simulink model "power_KundurTwoAreaSystem_0"  (R2021b)
settings: Solver=FixedStepDiscrete  StartTime=0.0  StopTime=5  MaxStep=1/60  RelTol=1e-4
PreLoadFcn:
  | Ts=50e-6;
  | Tctrl=2*Ts;
  | PSSMODEL=1;
undefined symbols (not defined in the file or in its folder): D1, Delta
libraries: spsGenericPowerSystemStabilizerLib x8, spsThreePhaseVIMeasurementLib x6, spsLoadFlowBusLib x6, spsThreePhaseParallelRLCLoadLib x4, spsThreePhasePISectionLineLib x4, spsSynchronousMachinepuStandardLib x4, spsExcitationSystemLib x4, spsSteamTurbineandGovernorLib x4, spsThreePhaseSeriesRLCLoadLib x4, spsThreePhaseTransformerTwoWindingsLib x4, spsThreePhaseBreakerLib x2, spsDistributedParametersLineLib x2
(part 1 of 2)
settings Model: ARTEMISmethode_block_infos=$$__separator__$$  Creator=The MathWorks, Inc.  LastModifiedBy=Pavel
settings SolverCC: AlgebraicLoopSolver=TrustRegion
settings DataIOCC: SaveOutput=off  SignalLogging=off  DSMLogging=off  SaveTime=off  ReturnWorkspaceOutputs=off  TimeSaveName=t  SignalLoggingName=sigsOut
settings OptimizationCC: BlockReduction=off  BooleanDataType=off  OptimizeBlockIOStorage=off  BufferReuse=off  GlobalBufferReuse=off  ExpressionFolding=off  ExpressionDepthLimit=2147483647  LocalBlockOutputs=off  InitFltsAndDblsToZero=on  LifeSpan=inf  OptimizeDataStoreBuffers=off  BusAssignmentInplaceUpdate=off
settings DebuggingCC: SaveWithParameterizedLinksMsg=none  SignalResolutionControl=TryResolveAllWithWarning  MultiTaskDSMMsg=warning  MultiTaskCondExecSysMsg=none  FcnCallInpInsideContextMsg=warning  UnconnectedOutputMsg=none  StateNameClashWarn=warning  SFUnexpectedBacktrackingDiag=warning  SFNoUnconditionalDefaultTransitionDiag=warning  SFExecutionAtInitializationDiag=none  SFMachineParentedDataDiag=warning  ArithmeticOperatorsInVariantConditions=warning
settings HardwareCC: ProdBitPerPointer=32  ProdBitPerSizeT=32  ProdBitPerPtrDiffT=32  ProdLargestAtomicFloat=None  ProdIntDivRoundTo=Undefined  ProdEndianess=Unspecified  ProdWordSize=32  ProdHWDeviceType=32-bit Generic  TargetBitPerPointer=64  TargetBitPerSizeT=64  TargetBitPerPtrDiffT=64  TargetLongLongMode=on  TargetIntDivRoundTo=Zero  TargetEndianess=LittleEndian  TargetWordSize=64  TargetHWDeviceType=MATLAB Host  ProdEqTarget=off
settings ModelReferenceCC: PropagateSignalLabelsOutOfModel=off
settings SFSimCC: SimUseLocalCustomCode=off  CustomCodeUndefinedFunction=UseInterfaceOnly
settings RTWCC: RTWUseLocalCustomCode=off
settings CodeAppCC: StateflowObjectComments=on
settings GRTTargetCC: TargetFcnLib=ansi_tfl_tmw.mat  TargetLangStandard=C89/C90 (ANSI)  CombineOutputUpdateFcns=off  GRTInterface=on
settings ConfigComp: CovMetricSettings=dw  CovSaveCumulativeToWorkspaceVar=on  CovSaveSingleToWorkspaceVar=on  CovExternalEMLEnable=off  CovSFcnEnable=off
settings SimscapeCC: SimscapeNormalizeSystem=off  SimscapeNominalValues={1, 'bar'; 1, 'cm^3/s'; 1, 'bar*kg/s'; 1, 'kJ/kg'; 1, 'kW'; }

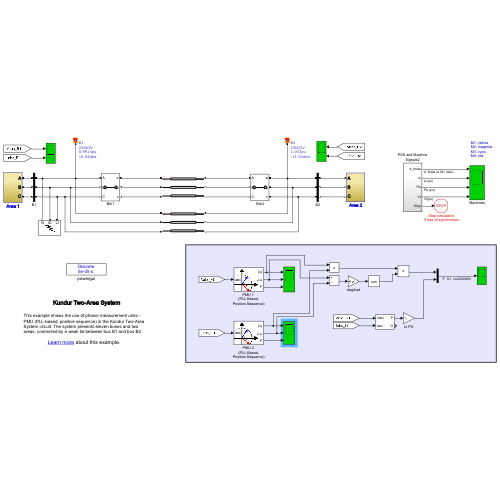
[thumbnail: Simulink's stored preview of the top-level diagram]
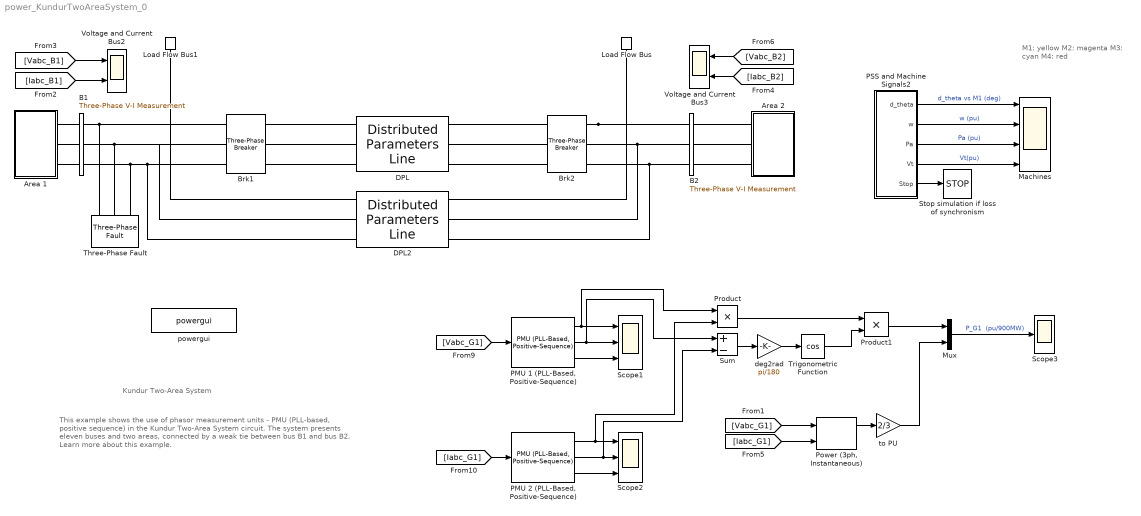
== system power_KundurTwoAreaSystem_0 ==
  note: This example shows the use of phasor measurement units - PMU (PLL-based, positive sequence) in the Kundur Two-Area System circuit. The system presents eleven buses and two areas, connected by a weak tie between bus B1 and bus B2.
      |
      | Learn more about this example.
  note: M1: yellow
      | M2: magenta
      | M3: cyan
      | M4: red
  note: Kundur Two-Area System
  " Brk2" : spsThreePhaseBreakerLib/Three-Phase Breaker  InitialState=closed  SwitchA=on  SwitchB=on  SwitchC=on  SwitchTimes=[2+12]*100  External=off  BreakerResistance=0.001  SnubberResistance=1e6  SnubberCapacitance=0  Measurements=None
      settings: AttributesFormatString=\n
  Area 1 : Subsystem
  Area 2 : Subsystem
  B1 : spsThreePhaseVIMeasurementLib/Three-Phase V-I Measurement  VoltageMeasurement=phase-to-ground  SetLabelV=on  LabelV=Vabc_B1  Vpu=on  VpuLL=off  CurrentMeasurement=yes  SetLabelI=on  LabelI=Iabc_B1  Ipu=off  Pbase=100e6  Vbase=230e3  OutputType=Complex  PhasorSimulation=off  PSBequivalent=0
  B2 : spsThreePhaseVIMeasurementLib/Three-Phase V-I Measurement  VoltageMeasurement=phase-to-ground  SetLabelV=on  LabelV=Vabc_B2  Vpu=off  VpuLL=off  CurrentMeasurement=yes  SetLabelI=on  LabelI=Iabc_B2  Ipu=off  Pbase=100e6  Vbase=500e3  OutputType=Complex  PhasorSimulation=off  PSBequivalent=0
  Brk1 : spsThreePhaseBreakerLib/Three-Phase Breaker  InitialState=closed  SwitchA=off  SwitchB=off  SwitchC=off  SwitchTimes=[2+12]  External=off  BreakerResistance=0.001  SnubberResistance=inf  SnubberCapacitance=0  Measurements=None
      settings: AttributesFormatString=\n
  DPL : spsDistributedParametersLineLib/Distributed Parameters Line  Phases=3  Length=220  Frequency=60  Resistance=[0.0001*529 1.61]  Inductance=[0.001*529/(377) 0.0061]  Capacitance=[0.00175/529/(377) 5.2489e-9]  x1=[-0.00125 5.00401938795932e-05 67714.9475638958 -217904.118381786;-0.0012 4.86656945364756e-05 71810.0841570275 -216589.0762183;-0.00115 4.72739045038167e-05 75879.7069691904 -215197.080987348;-0.0011 4.58653182779878e-05 79922.3700827773 -213728.627258207;-0.00105 4.44404363229678e-05 83936.6371588335 -212184.236765496;-0.001 4.29997648925308e-05 87921.0819473815 -210564.458223802;-0.00095 4.15438158503758e-05 91874.2887941601 -208869.867132729;-0.0009 4.0073106488265e-05 95794.8531436005 -207101.065572422;-0.00085 3.85881593422317e-05 99681.3820378574 -205258.681989653;-0.0008 3.70895020069262e-05 103532.494611721 -203343.370974537;-0.00075 3.55776669481637e-05 107346.822583231 -201355.813027957;-0.0007 3.40531913137418e-05 111123.010739822 -199296.714319788;-0.00065 3.25166167425944e-05 114859.717419823 -197166.806437996;-0.0006 3.096848917235e-05 118555.614989142 -194966.846128709;-0.00055 2.94093586453629e-05 122209.390312972 -192697.61502735;-0.0005 2.78397791132851e-05 125819.745222338 -190359.919380925;-0.00045 2.62603082402508e-05 129385.396975333 -187954.589761565;-0.0004 2.46715072047404e-05 132905.078712866 -185482.48077143;-0.00035 2.30739405001963e-05 136377.539908775 -182944.470739074;-0.0003 2.14681757344618e-05 139801.546814133 -180341.461407377;-0.00025 1.98547834281122e-05 143175.882895589 -177674.377613158;-0.0002 1.82343368117514e-05 146499.349267601 -174944.166958591;-0.00015 1.66074116223463e-05 149770.765118393 -172151.799474521;-0.0001 1.497458589867e-05 152988.968129489 -169298.267275818;-5e-05 1.33364397759271e-05 156152.814888683 -166384.584208886]  x2=[-0.00125 6.64238273339932e-05 -37054.7346638215 -227714.949033752;-0.0012 6.59450869998179e-05 -32756.0754824648 -228372.906194685;-0.00115 6.54429166902368e-05 -28445.7782234611 -228949.723549471;-0.0011 6.49174948239698e-05 -24125.3743149025 -229445.196157652;-0.00105 6.43690080809043e-05 -19796.3987757256 -229859.147980168;-0.001 6.37976513357682e-05 -15460.3896703266 -230191.431941908;-0.00095 6.32036275888925e-05 -11118.8875620942 -230441.929983962;-0.0009 6.25871478940861e-05 -6773.43496605488 -230610.55310557;-0.00085 6.1948431283649e-05 -2425.57580082464 -230697.241395739;-0.0008 6.12877046905515e-05 1923.14515993797 -230701.964054532;-0.00075 6.06052028678062e-05 6271.18283638253 -230624.719404011;-0.0007 5.99011683050607e-05 10616.9923914263 -230465.534888833;-0.00065 5.91758511424429e-05 14959.0297796275 -230224.467066497;-0.0006 5.84295090816871e-05 19295.7522957771 -229901.601587254;-0.00055 5.76624072945735e-05 23625.6191230151 -229497.05316367;-0.0005 5.68748183287145e-05 27947.0918802748 -229010.965529875;-0.00045 5.60670220107194e-05 32258.6351688628 -228443.51139049;-0.0004 5.52393053467737e-05 36558.7171179787 -227794.892359268;-0.00035 5.43919624206668e-05 40845.8099289812 -227065.338887463;-0.0003 5.35252942893056e-05 45118.390418208 -226255.110181951;-0.00025 5.26396088757503e-05 49374.9405581558 -225364.49411313;-0.0002 5.17352208598112e-05 53613.9480168279 -224393.807112651;-0.00015 5.0812451566244e-05 57833.9066950588 -223343.394060983;-0.0001 4.98716288505848e-05 62033.3172616238 -222213.628164881;-5e-05 4.89130869826646e-05 66210.6876859448 -221004.910824788]  x3=[-0.00125 5.68511441714353e-09 -84.0164435730609 325.429221773661;-0.0012 5.94435553554912e-09 -90.1353537591281 323.787794066755;-0.00115 6.20148465273767e-09 -96.2222392831948 322.03132609837;-0.0011 6.4564104119582e-09 -102.274937503818 320.160441933214;-0.00105 6.70904223930233e-09 -108.29129792614 318.175806287519;-0.001 6.95929037588473e-09 -114.269182965951 316.078124292883;-0.00095 7.20706590973406e-09 -120.20646870916 313.868141245729;-0.0009 7.45228080738296e-09 -126.101045666414 311.54664234251;-0.00085 7.69484794514591e-09 -131.950819522587 309.114452400733;-0.0008 7.93468114007387e-09 -137.753711880884 306.572435565903;-0.00075 8.17169518057469e-09 -143.50766100128 303.921495004497;-0.0007 8.40580585668834e-09 -149.210622533051 301.162572583075;-0.00065 8.63692999000634e-09 -154.86057024112 298.296648533634;-0.0006 8.86498546322466e-09 -160.455496725969 295.324741105345;-0.00055 9.08989124931957e-09 -165.993414136859 292.247906202764;-0.0005 9.31156744033618e-09 -171.472354878104 289.067237010682;-0.00045 9.52993527577937e-09 -176.890372308146 285.783863605718;-0.0004 9.74491717059699e-09 -182.245541431192 282.398952554809;-0.00035 9.95643674274547e-09 -187.535959581151 278.913706500733;-0.0003 1.0164418840328e-08 -192.759747097645 275.329363734817;-0.00025 1.03687895682956e-08 -197.915047993843 271.64719775698;-0.0002 1.05694763147019e-08 -203.000030615886 267.86851682326;-0.00015 1.07664077765013e-08 -208.012888293659 263.994663481001;-0.0001 1.09595139848833e-08 -212.951839982699 260.027014091848;-5e-05 1.11487263301314e-08 -217.815130896989 255.966978342738]  x4=[-0.00125 9.68423697480985e-08 -1.92606776170441 -1426.66433970826;-0.0012 9.56520018607397e-08 24.9647096485138 -1426.44709548488;-0.00115 9.44276492725781e-08 51.8466172162664 -1425.72304140067;-0.0011 9.31697469902584e-08 78.7101039277956 -1424.49243470859;-0.00105 9.18787419404718e-08 105.545625314187 -1422.75571263736;-0.001 9.05550928111652e-08 132.343646842472 -1420.51349223604;-0.00095 8.91992698885716e-08 159.094647303204 -1417.76657015487;-0.0009 8.78117548901194e-08 185.789122193297 -1414.51592236219;-0.00085 8.63930407932808e-08 212.417587092931 -1410.76270379768;-0.0008 8.49436316604189e-08 238.970581035323 -1406.50824796203;-0.00075 8.34640424596973e-08 265.43866986816 -1401.75406644312;-0.0007 8.19547988821136e-08 291.81244960551 -1396.50184837903;-0.00065 8.04164371547246e-08 318.082549769014 -1390.75345985782;-0.0006 7.88495038501268e-08 344.239636717173 -1384.51094325456;-0.00055 7.72545556922623e-08 370.274416961545 -1377.77651650567;-0.0005 7.56321593586171e-08 396.177640468675 -1370.55257232091;-0.00045 7.39828912788831e-08 421.940103946593 -1362.84167733325;-0.0004 7.23073374301561e-08 447.552654114697 -1354.64657118697;-0.00035 7.060609312874e-08 473.006190955868 -1345.97016556426;-0.0003 6.88797628186346e-08 498.291670949668 -1336.81554315071;-0.00025 6.71289598567788e-08 523.400110285454 -1327.18595654009;-0.0002 6.53543062951283e-08 548.322588054286 -1317.08482707867;-0.00015 6.35564326596434e-08 573.050249418486 -1306.51574364963;-0.0001 6.17359777262661e-08 597.574308757714 -1295.48246139801;-5e-05 5.98935882939657e-08 621.886052790461 -1283.98890039645]  x5=0.00124486354111605  V1=ones(3,3)  V2=ones(3,3)  I1=ones(3,3)  I2=ones(3,3)  nHarmo=1  Measurements=None  Decoupling=off  VsMag0=0  VrMag0=0  VsAngle0=0  VrAngle0=0  IsMag0=0  IrMag0=0  IsAngle0=0  IrAngle0=0
      settings: SourceProductBaseCode=PS
  DPL2 : spsDistributedParametersLineLib/Distributed Parameters Line  Phases=3  Length=220  Frequency=60  Resistance=[0.0001*529 1.61]  Inductance=[0.001*529/(377) 0.0061]  Capacitance=[0.00175/529/(377) 5.2489e-9]  x1=[-0.00125 5.0041693650628e-05 67715.2009241801 -217904.989560214;-0.0012 4.86670938538175e-05 71810.3538926926 -216589.942466454;-0.00115 4.72752028702947e-05 75879.9929844005 -215197.941997455;-0.0011 4.58665152322987e-05 79922.6722759125 -213729.482724354;-0.00105 4.44415314398394e-05 83936.9554225262 -212185.08638374;-0.001 4.30007577828731e-05 87921.416168554 -210565.301692277;-0.00095 4.15447061614197e-05 91874.6388540653 -208870.704151755;-0.0009 4.00738939036873e-05 95795.2189178637 -207101.89584461;-0.00085 3.85888435822674e-05 99681.7633965208 -205259.505220012;-0.0008 3.70900828284681e-05 103532.89141929 -203344.186870577;-0.00075 3.55781441448486e-05 107347.234698721 -201356.621299794;-0.0007 3.4053564716024e-05 111123.438016811 -199297.514680246;-0.00065 3.25168862178058e-05 114860.159706501 -197167.598602711;-0.0006 3.09686546247475e-05 118556.072128367 -194967.629816229;-0.00055 2.94094200161619e-05 122209.862142324 -192698.389959235;-0.0005 2.78397363806809e-05 125820.23157418 -190360.685281844;-0.00045 2.62601614194262e-05 129385.897676864 -187955.346359398;-0.0004 2.46712563478599e-05 132905.593586191 -185483.227797362;-0.00035 2.30735856963883e-05 136378.068770962 -182945.20792769;-0.0003 2.14677171097865e-05 139802.089477278 -180342.188496756;-0.00025 1.98542211455166e-05 143176.439166888 -177675.09434497;-0.0002 1.82336710710118e-05 146499.918949413 -174944.873078184;-0.00015 1.66066426599974e-05 149771.348008313 -172152.494731014;-0.0001 1.49737139879203e-05 152989.564020418 -169298.951422191;-5e-05 1.33354652265625e-05 156153.423568905 -166385.257002064]  x2=[-0.00125 6.64214580413413e-05 -37054.8247033456 -227714.066792769;-0.0012 6.59426867546337e-05 -32756.1821348863 -228372.025807605;-0.00115 6.54404863453161e-05 -28445.9014508868 -228948.845329093;-0.0011 6.49150352428025e-05 -24125.5140735503 -229444.320416002;-0.00105 6.43665201373679e-05 -19796.55501594 -229858.275028394;-0.001 6.37951359138171e-05 -15460.5623365962 -230190.562090165;-0.00095 6.32010855822443e-05 -11119.0765930715 -230441.063541305;-0.0009 6.25845802059036e-05 -6773.64029457802 -230609.690379841;-0.00085 6.19458388262195e-05 -2425.7973539414 -230696.382693461;-0.0008 6.12850883849629e-05 1922.90746094438 -230701.109680798;-0.00075 6.06025636436193e-05 6270.92907596541 -230623.869662375;-0.0007 5.98985070999794e-05 10616.7226597455 -230464.690081204;-0.00065 5.91731689019807e-05 14958.7441725174 -230223.627493033;-0.0006 5.84268067588311e-05 19295.4509147126 -229900.76754625;-0.00055 5.76596858494463e-05 23625.3020750754 -229496.224951457;-0.0005 5.68720787282325e-05 27946.7592781056 -229010.143440713;-0.00045 5.60642652282497e-05 32258.2871306361 -228442.695716463;-0.0004 5.5236532361788e-05 36558.3537673507 -227794.083390181;-0.00035 5.43891742183934e-05 40845.4313950486 -227064.53691074;-0.0003 5.35224918603794e-05 45117.9968354623 -226254.315482529;-0.00025 5.26367932158611e-05 49374.5320664349 -225363.706973363;-0.0002 5.17323929693495e-05 53613.5247612671 -224393.027812206;-0.00015 5.08096124499458e-05 57833.4688260387 -223342.622876741;-0.0001 4.98687795171746e-05 62032.8649347172 -222212.86537084;-5e-05 4.8910228444497e-05 66210.2210618613 -221004.156691966]  x3=[-0.00125 5.67985394464599e-09 -84.0015107882101 325.431384816722;-0.0012 5.93900034567544e-09 -90.1204643958681 323.79023818478;-0.00115 6.19603664816132e-09 -96.2073986316455 322.034050422975;-0.0011 6.45087152832926e-09 -102.260150836792 320.163445496458;-0.00105 6.70341444455978e-09 -108.27657049727 318.179088022253;-0.001 6.95357566955725e-09 -114.254520007822 316.08168303312;-0.00095 7.20126632222959e-09 -120.191875431451 313.871975727066;-0.0009 7.44639839926732e-09 -126.086527254048 311.550751202575;-0.00085 7.6888848064107e-09 -131.936381133887 309.118834179667;-0.0008 7.9286393893939e-09 -137.73935864574 306.577088706881;-0.00075 8.16557696455519e-09 -143.493398019328 303.92641785428;-0.0007 8.39961334910234e-09 -149.196454871861 301.167763392597;-0.00065 8.6306653910223e-09 -154.846502934394 298.302105458627;-0.0006 8.85865099862476e-09 -160.441534771754 295.330462206988;-0.00055 9.08348916970892e-09 -165.979562495772 292.253889448377;-0.0005 9.30510002034319e-09 -171.458618471566 289.073480274447;-0.00045 9.52340481324757e-09 -176.876756016637 285.790364669433;-0.0004 9.73832598576861e-09 -182.232050092516 282.405709108676;-0.00035 9.9497871774371e-09 -187.522597988715 278.920716144182;-0.0003 1.01577132570985e-08 -192.746519998761 275.336623977355;-0.00025 1.03620303496069e-08 -197.901960088036 271.654706019076;-0.0002 1.0562665862072e-08 -202.987086553225 267.876270437266;-0.00015 1.07595485096518e-08 -208.00009267311 264.002659692093;-0.0001 1.09526083408789e-08 -212.939197350484 260.035250059011;-5e-05 1.11417767625146e-08 -217.802645744975 255.975451139772]  x4=[-0.00125 9.68486646687031e-08 -1.94059700386609 -1426.66653467617;-0.0012 9.5658299002309e-08 24.9502243580123 -1426.44956391594;-0.00115 9.44339463977677e-08 51.8321810239799 -1425.72578241787;-0.0011 9.31760418617297e-08 78.6957219628346 -1424.49544733806;-0.00105 9.18850323216868e-08 105.531302686395 -1422.75899580871;-0.001 9.05613764671816e-08 132.329388640611 -1420.51704478279;-0.00095 8.92055445868362e-08 159.080458593144 -1417.77039081481;-0.0009 8.78180184012618e-08 185.77500801622 -1414.52000977786;-0.00085 8.63992908919053e-08 212.403552463537 -1410.76705651684;-0.0008 8.49498661258954e-08 238.956630940049 -1406.51286443818;-0.00075 8.34702590769497e-08 265.424809263407 -1401.75894503605;-0.0007 8.19609954424075e-08 291.798683415886 -1396.5069873554;-0.00065 8.04226114564516e-08 318.068882885582 -1390.75885739177;-0.0006 7.88556536995869e-08 344.22607399571 -1384.51659742837;-0.00055 7.72606789044433e-08 370.260963220821 -1377.78242531044;-0.0005 7.56382537579707e-08 396.164300488741 -1370.55873365728;-0.00045 7.39889547000985e-08 421.92688246708 -1362.84808901212;-0.0004 7.23133677189284e-08 447.539555833133 -1354.6532309303;-0.00035 7.06120881425364e-08 472.993220526012 -1345.97707100588;-0.0003 6.88857204274552e-08 498.27883297985 -1336.82269183715;-0.00025 6.71348779439135e-08 523.387409336944 -1327.19334593145;-0.0002 6.53601827579091e-08 548.310028639672 -1317.09245454953;-0.00015 6.3562265410191e-08 573.037836000067 -1306.52360649;-0.0001 6.17417646922319e-08 597.562045745918 -1295.49055681425;-5e-05 5.98993274192683e-08 621.873944542278 -1283.99722551229]  x5=0.00124486354111605  V1=ones(3,3)  V2=ones(3,3)  I1=ones(3,3)  I2=ones(3,3)  nHarmo=1  Measurements=None  Decoupling=off  VsMag0=0  VrMag0=0  VsAngle0=0  VrAngle0=0  IsMag0=0  IrMag0=0  IsAngle0=0  IrAngle0=0
      settings: SourceProductBaseCode=PS
  Load Flow Bus : spsLoadFlowBusLib/Load Flow Bus  LConnTagsString=a  Phases=single  Connectors=on one side  ID=B2  Vbase=230e3  Vref=1  Vangle=0  VLF=1.003  VLFb=1  VLFc=1  angleLF=-11.54  angleLFb=0  angleLFc=0
      settings: AttributesFormatString=%<ID>\n%<Vbase>V\n%<VLF>pu\n%<angleLF>deg.  SourceProductBaseCode=PS
  Load Flow Bus1 : spsLoadFlowBusLib/Load Flow Bus  LConnTagsString=a  Phases=single  Connectors=on one side  ID=B1  Vbase=230e3  Vref=1  Vangle=0  VLF=0.9914  VLFb=1  VLFc=1  angleLF=15.04  angleLFb=0  angleLFc=0
      settings: AttributesFormatString=%<ID>\n%<Vbase>V\n%<VLF>pu\n%<angleLF>deg.  SourceProductBaseCode=PS
  Machines : Scope  NumInputPorts=4
  Mux : Mux  Inputs=2
  "PMU 1 (PLL-Based, Positive-Sequence)" : spsPMUPLLBasedPositiveSequenceLib/PMU (PLL-Based, Positive-Sequence)  nominalFrequency=60  samplingRate=64  reportingFactor=1
      settings: SourceProductBaseCode=PS
  "PMU 2 (PLL-Based, Positive-Sequence)" : spsPMUPLLBasedPositiveSequenceLib/PMU (PLL-Based, Positive-Sequence)  nominalFrequency=60  samplingRate=64  reportingFactor=1
      settings: SourceProductBaseCode=PS
  PSS and Machine Signals2 : Subsystem
  "Power (3ph, Instantaneous)" : spsPower3phInstantaneousLib/Power (3ph, Instantaneous)
  Product : Product
  Product1 : Product
  Scope1 : Scope  NumInputPorts=3
  Scope2 : Scope  NumInputPorts=3
  Scope3 : Scope
  Stop simulation if loss of synchronism : Stop
  Sum : Sum  Inputs=+-
  Three-Phase Fault : spsThreePhaseFaultLib/Three-Phase Fault  InitialStates=0  FaultA=on  FaultB=on  FaultC=on  GroundFault=on  SwitchTimes=[2 2.1]  External=off  SwitchStatus=NaN  FaultResistance=0.001  GroundResistance=0.001  SnubberResistance=1e6  SnubberCapacitance=inf  Measurements=None
  Trigonometric Function : Trigonometry  Operator=cos
  Voltage and Current Bus2 : Scope  NumInputPorts=2
  Voltage and Current Bus3 : Scope  NumInputPorts=2
  deg2rad : Gain  Gain=pi/180
  powergui : spspowerguiLib/powergui  Priority=2  SimulationMode=Discrete  SampleTime=Ts  frequency=60  Iterations=50  frequencyindice=60  Pbase=100e6  ErrMax=1e-4  UnitsV=kV  UnitsW=MW  buscounter=0  FunctionMessages=off  echomessages=off  EnableUseOfTLC=off  CurrentSourceSwitches=off  DisableSnubberDevices=off  DisableRonSwitches=off  DisableVfSwitches=off  DisplayEquations=off  AutomaticDiscreteSolvers=off  SolverType=Tustin  Interpol=off  ExternalGateDelay=off  methode=off  Ts=0  x0status=blocks  SPID=off  SwTol=0  HookPort=off  NonlinearTolerance=1e-4  nMaxIteration=100  ContinueOnMaxIteration=off  RestoreLinks=warning  ResistiveCurrentMeasurement=off  Frange=logspace(0,3,50)  Ylog=off  Xlog=off  ShowGrid=off  save=off  variable=ZData  structure=0  ZoomFFT=on  StartTime=0.0  cycles=1  DisplayStyle=1  fundamental=60  FreqAxis=off  MaxFrequency=1000  frequencyindicesteady=1  RmsSteady=1  display=off
  to PU : Gain  Gain=2/3
  wires:
  [Iabc_B1] -> Voltage and Current Bus2/2
  [Vabc_B1] -> Voltage and Current Bus2/1
  [Iabc_B2] -> Voltage and Current Bus3/2
  [Vabc_B2] -> Voltage and Current Bus3/1
  PSS and Machine Signals2/1(d_theta) -> Machines/1  "d_theta vs M1 (deg)"
  PSS and Machine Signals2/2(w) -> Machines/2  "w (pu)"
  PSS and Machine Signals2/3(Pa) -> Machines/3  "Pa (pu)"
  PSS and Machine Signals2/4(Vt) -> Machines/4  "Vt(pu)"
  PSS and Machine Signals2/5(Stop) -> Stop simulation if loss of synchronism/1
  [Iabc_G1] -> "PMU 2 (PLL-Based, Positive-Sequence)"/1
  "PMU 2 (PLL-Based, Positive-Sequence)"/3 -> Scope2/3
  [Vabc_G1] -> "PMU 1 (PLL-Based, Positive-Sequence)"/1
  "PMU 1 (PLL-Based, Positive-Sequence)"/3 -> Scope1/3
  Product/1 -> Product1/1
  [Iabc_G1] -> "Power (3ph, Instantaneous)"/2
  "Power (3ph, Instantaneous)"/1 -> to PU/1
  "PMU 2 (PLL-Based, Positive-Sequence)"/1 -> Product/2, Scope2/1
  [Vabc_G1] -> "Power (3ph, Instantaneous)"/1
  "PMU 2 (PLL-Based, Positive-Sequence)"/2 -> Sum/2, Scope2/2
  deg2rad/1 -> Trigonometric Function/1
  "PMU 1 (PLL-Based, Positive-Sequence)"/1 -> Scope1/1, Product/1
  Trigonometric Function/1 -> Product1/2
  Product1/1 -> Mux/1
  Sum/1 -> deg2rad/1
  to PU/1 -> Mux/2
  "PMU 1 (PLL-Based, Positive-Sequence)"/2 -> Sum/1, Scope1/2
  Mux/1 -> Scope3/1  "P_G1  (pu/900MW)"
  connections:
  " Brk2"/RConn1 -- DPL2/RConn1 -- B2/LConn1 -- Load Flow Bus/LConn1
  " Brk2"/RConn2 -- DPL2/RConn2 -- B2/LConn2
  " Brk2"/RConn3 -- DPL2/RConn3 -- B2/LConn3
  B2/RConn3 -- Area 2/LConn3
  B2/RConn2 -- Area 2/LConn2
  Area 2/LConn1 -- B2/RConn1
  Area 1/RConn3 -- B1/LConn3
  Area 1/RConn2 -- B1/LConn2
  Area 1/RConn1 -- B1/LConn1
  " Brk2"/LConn3 -- DPL/RConn3
  " Brk2"/LConn2 -- DPL/RConn2
  DPL/RConn1 -- " Brk2"/LConn1
  Brk1/RConn3 -- DPL/LConn3
  Brk1/RConn2 -- DPL/LConn2
  Brk1/RConn1 -- DPL/LConn1
  DPL2/LConn3 -- B1/RConn3 -- Three-Phase Fault/LConn3 -- Brk1/LConn3
  DPL2/LConn2 -- Brk1/LConn2 -- Three-Phase Fault/LConn2 -- B1/RConn2
  DPL2/LConn1 -- Brk1/LConn1 -- Load Flow Bus1/LConn1 -- Three-Phase Fault/LConn1 -- B1/RConn1

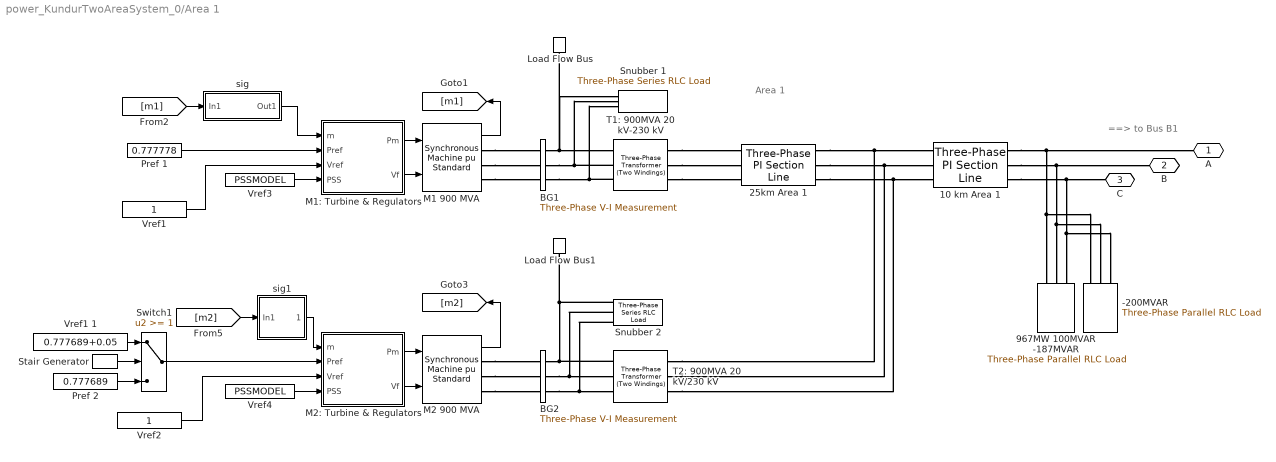
== system power_KundurTwoAreaSystem_0/Area 1 ==
  note: Area 1
  note: ==> to Bus B1
  -200MVAR : spsThreePhaseParallelRLCLoadLib/Three-Phase Parallel RLC Load  LConnTagsString=A|B|C  Configuration=Y (grounded)  NominalVoltage=230e3  Vabc=[1e3 1e3 1e3]  Vabcp=[1e3 1e3 1e3]  NominalFrequency=60  UnbalancedPower=off  ActivePower=0  InductivePower=0  CapacitivePower=200e6  Pabc=[10e3 9e3 11e3]  QLabc=[100 90 110]  QCabc=[100 90 110]  Pabcp=[10e3 9e3 11e3]  QLabcp=[100 90 110]  QCabcp=[100 90 110]  Measurements=None  LoadType=constant Z
  10 km Area 1 : spsThreePhasePISectionLineLib/Three-Phase PI Section Line  LConnTagsString=a|b|c  RConnTagsString=A|B|C  Length=10  Frequency=60  Resistances=[0.0001*529 1.61]  Inductances=[0.001*529/(377) 0.0061]  Capacitances=[0.00175/529/(377) 5.2489e-9]
  25km Area 1 : spsThreePhasePISectionLineLib/Three-Phase PI Section Line  LConnTagsString=a|b|c  RConnTagsString=A|B|C  Length=25  Frequency=60  Resistances=[0.0001*529 1.61]  Inductances=[0.001*529/(377) 0.0061]  Capacitances=[0.00175/529/(377) 5.2489e-9]
  967MW 100MVAR -187MVAR : spsThreePhaseParallelRLCLoadLib/Three-Phase Parallel RLC Load  LConnTagsString=A|B|C  Configuration=Y (grounded)  NominalVoltage=230e3  Vabc=[1e3 1e3 1e3]  Vabcp=[1e3 1e3 1e3]  NominalFrequency=60  UnbalancedPower=off  ActivePower=967e6  InductivePower=100e6  CapacitivePower=187e6  Pabc=[10e3 9e3 11e3]  QLabc=[100 90 110]  QCabc=[100 90 110]  Pabcp=[10e3 9e3 11e3]  QLabcp=[100 90 110]  QCabcp=[100 90 110]  Measurements=None  LoadType=constant Z
  BG1 : spsThreePhaseVIMeasurementLib/Three-Phase V-I Measurement  VoltageMeasurement=phase-to-ground  SetLabelV=on  LabelV=Vabc_G1  Vpu=on  VpuLL=off  CurrentMeasurement=yes  SetLabelI=on  LabelI=Iabc_G1  Ipu=on  Pbase=900e6  Vbase=20e3  OutputType=Complex  PhasorSimulation=off  PSBequivalent=0
  BG2 : spsThreePhaseVIMeasurementLib/Three-Phase V-I Measurement  VoltageMeasurement=no  SetLabelV=on  LabelV=Vabc_G2  Vpu=on  VpuLL=off  CurrentMeasurement=no  SetLabelI=on  LabelI=Iabc_G2  Ipu=on  Pbase=900e6  Vbase=20e3  OutputType=Complex  PhasorSimulation=off  PSBequivalent=0
  Load Flow Bus : spsLoadFlowBusLib/Load Flow Bus  LConnTagsString=a  Phases=single  Connectors=on one side  ID=M1_Area1  Vbase=20e3  Vref=1  Vangle=0  VLF=1  VLFb=1  VLFc=1  angleLF=10.19  angleLFb=0  angleLFc=0
      settings: AttributesFormatString=%<ID>\n%<Vbase>V\n%<VLF>pu\n%<angleLF>deg.  SourceProductBaseCode=PS
  Load Flow Bus1 : spsLoadFlowBusLib/Load Flow Bus  LConnTagsString=a  Phases=single  Connectors=on one side  ID=M2_Area1  Vbase=20e3  Vref=1  Vangle=0  VLF=1  VLFb=1  VLFc=1  angleLF=0  angleLFb=0  angleLFc=0
      settings: AttributesFormatString=%<ID>\n%<Vbase>V\n%<VLF>pu\n%<angleLF>deg.  SourceProductBaseCode=PS
  M1 900 MVA : spsSynchronousMachinepuStandardLib/Synchronous Machine pu Standard  PresetModel=No  MechanicalLoad=Mechanical power Pm  ShowDetailedParameters=on  RotorType=Round  Units=per unit standard parameters  MeasurementBus=off  NominalParameters="[900E6  20000   60 ]"  Reactances1=[1.8 .3 .25 1.7 .55 .25 .2]  Reactances2=[ 1.305, 0.296, 0.252, 0.474, 0.243, 0.18 ]  dAxisTimeConstants=Open-circuit  qAxisTimeConstants=Open-circuit  TimeConstants1=[]  TimeConstants2=[8 .03 .4 .05]  TimeConstants3=[]  TimeConstants4=[]  TimeConstants5=[ 1.01, 0.053, 0.1 ]  TimeConstants6=[]  TimeConstants7=[]  TimeConstants8=[]  StatorResistance=0.0025  Mechanical="[ 6.5 0  4]"  PolePairs=4  InitialConditions=[0 -31.4247 0.784453 0.784453 0.784453 2.7401 -117.26 122.74 1.83395]  SetSaturation=off  Saturation=[0.6404,0.7127,0.8441,0.9214,0.9956,1.082,1.19,1.316,1.457;0.7,0.7698,0.8872,0.9466,0.9969,1.046,1.1,1.151,1.201]  LoadFlowParameters=[1 700000000 0 0 0]  TsPowergui=0  TsBlock=-1  IterativeModel=Trapezoidal non iterative  IterativeDiscreteModel=Trapezoidal non iterative  BusType=PV  Pref=700000000  Qref=0  Qmin=-inf  Qmax=inf  PLF=0  QLF=0
      settings: SourceProductBaseCode=PS
  M1: Turbine & Regulators : Subsystem
  M2 900 MVA : spsSynchronousMachinepuStandardLib/Synchronous Machine pu Standard  PresetModel=No  MechanicalLoad=Mechanical power Pm  ShowDetailedParameters=on  RotorType=Round  Units=per unit standard parameters  MeasurementBus=off  NominalParameters="[900E6  20000   60 ]"  Reactances1=[1.8 .3 .25 1.7 .55 .25 .2]  Reactances2=[ 1.305, 0.296, 0.252, 0.474, 0.243, 0.18 ]  dAxisTimeConstants=Open-circuit  qAxisTimeConstants=Open-circuit  TimeConstants1=[]  TimeConstants2=[8 .03 .4 .05]  TimeConstants3=[]  TimeConstants4=[]  TimeConstants5=[ 1.01, 0.053, 0.1 ]  TimeConstants6=[]  TimeConstants7=[]  TimeConstants8=[]  StatorResistance=0.0025  Mechanical="[ 6.5 0  4]"  PolePairs=4  InitialConditions=[0 -42.8075 0.788608 0.788608 0.788608 -9.54571 -129.546 110.454 1.86756]  SetSaturation=off  Saturation=[0.6404,0.7127,0.8441,0.9214,0.9956,1.082,1.19,1.316,1.457;0.7,0.7698,0.8872,0.9466,0.9969,1.046,1.1,1.151,1.201]  LoadFlowParameters=[2 700000000 0 0 0]  TsPowergui=0  TsBlock=-1  IterativeModel=Trapezoidal non iterative  IterativeDiscreteModel=Trapezoidal non iterative  BusType=swing  Pref=0  Qref=0  Qmin=-inf  Qmax=inf  PLF=0  QLF=0
      settings: SourceProductBaseCode=PS
  M2: Turbine & Regulators : Subsystem
  Pref 1 : Constant  Value=0.777778
  Pref 2 : Constant  Value=0.777689
  Snubber 1 : spsThreePhaseSeriesRLCLoadLib/Three-Phase Series RLC Load  LConnTagsString=A|B|C  Configuration=Y (grounded)  NominalVoltage=20000  Vabc=[1e3 1e3 1e3]  Vabcp=[1e3 1e3 1e3]  NominalFrequency=60  UnbalancedPower=off  ActivePower=1e6  InductivePower=0  CapacitivePower=1e7  Pabc=[10e3 9e3 11e3]  QLabc=[100 90 110]  QCabc=[100 90 110]  Pabcp=[10e3 9e3 11e3]  QLabcp=[100 90 110]  QCabcp=[100 90 110]  Measurements=None  LoadType=constant Z
  Snubber 2 : spsThreePhaseSeriesRLCLoadLib/Three-Phase Series RLC Load  LConnTagsString=A|B|C  Configuration=Y (grounded)  NominalVoltage=20000  Vabc=[1e3 1e3 1e3]  Vabcp=[1e3 1e3 1e3]  NominalFrequency=60  UnbalancedPower=off  ActivePower=1e6  InductivePower=0  CapacitivePower=1e7  Pabc=[10e3 9e3 11e3]  QLabc=[100 90 110]  QCabc=[100 90 110]  Pabcp=[10e3 9e3 11e3]  QLabcp=[100 90 110]  QCabcp=[100 90 110]  Measurements=None  LoadType=constant Z
  Stair Generator : spsStairGeneratorLib/Stair Generator  t=[0 15 20]  e=[0 1 0 ]  Ts=0
  Switch1 : Switch  Threshold=1  InputSameDT=on
  T1: 900MVA 20 kV-230 kV : spsThreePhaseTransformerTwoWindingsLib/Three-Phase Transformer (Two Windings)  Winding1Connection=Delta (D1)  Winding2Connection=Yg  CoreType=Three single-phase transformers  SetSaturation=off  Hysteresis=off  DataFile='hysteresis'  SetInitialFlux=off  Measurements=None  UNITS=pu  NominalPower="[ 900e6   60 ]"  Winding1="[ 20e3  1e-6   0  ]"  Winding2="[ 230e3  1e-6   0.15 ]"  Rm=500  Lm=500  L0=0.5  Saturation="[ 0,0  ;  0.005,1.2  ;  1.0,1.4 ]"  InitialFluxes=[ 0.8 , -0.8 , 0.7 ]  BreakLoop=off  DiscreteSolver=Trapezoidal iterative  DataType=off  TransfoNumber=0
  T2: 900MVA 20 kV/230 kV : spsThreePhaseTransformerTwoWindingsLib/Three-Phase Transformer (Two Windings)  Winding1Connection=Delta (D1)  Winding2Connection=Yg  CoreType=Three single-phase transformers  SetSaturation=off  Hysteresis=off  DataFile='hysteresis'  SetInitialFlux=off  Measurements=None  UNITS=pu  NominalPower=[ 900e6 60 ]  Winding1="[ 20e3 1e-6  0.0]"  Winding2=[ 230e3 1e-6 0.15]  Rm=500  Lm=500  L0=0.5  Saturation="[ 0,0  ;  0.005,1.2  ;  1.0,1.4 ]"  InitialFluxes=[ 0.8 , -0.8 , 0.7 ]  BreakLoop=off  DiscreteSolver=Trapezoidal iterative  DataType=off  TransfoNumber=0
  Vref1 : Constant
  Vref1 1 : Constant  Value=0.777689+0.05
  Vref2 : Constant
  Vref3 : Constant  Value=PSSMODEL
  Vref4 : Constant  Value=PSSMODEL
  sig : Subsystem
  sig1 : Subsystem
  " A" : PMIOPort  Side=Right
  " B" : PMIOPort  Port=2  Side=Right
  " C" : PMIOPort  Port=3  Side=Right
  wires:
  Pref 1/1 -> M1: Turbine & Regulators/2(Pref)
  Vref2/1 -> M2: Turbine & Regulators/3(Vref)
  Vref4/1 -> M2: Turbine & Regulators/4(PSS)
  sig/1(Out1) -> M1: Turbine & Regulators/1(m)
  M1 900 MVA/1 -> [m1]
  M2 900 MVA/1 -> [m2]
  [m1] -> sig/1(In1)
  Vref3/1 -> M1: Turbine & Regulators/4(PSS)
  sig1/1(Out1) -> M2: Turbine & Regulators/1(m)
  [m2] -> sig1/1(In1)
  Stair Generator/1 -> Switch1/2
  Pref 2/1 -> Switch1/3
  Vref1 1/1 -> Switch1/1
  Switch1/1 -> M2: Turbine & Regulators/2(Pref)
  Vref1/1 -> M1: Turbine & Regulators/3(Vref)
  M1: Turbine & Regulators/1(Pm) -> M1 900 MVA/1
  M1: Turbine & Regulators/2(Vf) -> M1 900 MVA/2
  M2: Turbine & Regulators/2(Vf) -> M2 900 MVA/2
  M2: Turbine & Regulators/1(Pm) -> M2 900 MVA/1
  connections:
  T1: 900MVA 20 kV-230 kV/RConn1 -- 25km Area 1/LConn1
  T1: 900MVA 20 kV-230 kV/RConn2 -- 25km Area 1/LConn2
  Snubber 2/LConn1 -- T2: 900MVA 20 kV/230 kV/LConn1 -- BG2/RConn1 -- Load Flow Bus1/LConn1
  Snubber 2/LConn2 -- T2: 900MVA 20 kV/230 kV/LConn2 -- BG2/RConn2
  Snubber 2/LConn3 -- BG2/RConn3 -- T2: 900MVA 20 kV/230 kV/LConn3
  T1: 900MVA 20 kV-230 kV/RConn3 -- 25km Area 1/LConn3
  10 km Area 1/RConn1 -- " A"/RConn1 -- 967MW 100MVAR -187MVAR/LConn1 -- -200MVAR/LConn1
  10 km Area 1/RConn2 -- " B"/RConn1 -- 967MW 100MVAR -187MVAR/LConn2 -- -200MVAR/LConn2
  10 km Area 1/RConn3 -- " C"/RConn1 -- 967MW 100MVAR -187MVAR/LConn3 -- -200MVAR/LConn3
  Snubber 1/LConn1 -- Load Flow Bus/LConn1 -- T1: 900MVA 20 kV-230 kV/LConn1 -- BG1/RConn1
  T1: 900MVA 20 kV-230 kV/LConn2 -- Snubber 1/LConn2 -- BG1/RConn2
  T1: 900MVA 20 kV-230 kV/LConn3 -- Snubber 1/LConn3 -- BG1/RConn3
  25km Area 1/RConn2 -- 10 km Area 1/LConn2 -- T2: 900MVA 20 kV/230 kV/RConn2
  25km Area 1/RConn1 -- 10 km Area 1/LConn1 -- T2: 900MVA 20 kV/230 kV/RConn1
  25km Area 1/RConn3 -- 10 km Area 1/LConn3 -- T2: 900MVA 20 kV/230 kV/RConn3
  M1 900 MVA/RConn1 -- BG1/LConn1
  M1 900 MVA/RConn2 -- BG1/LConn2
  M1 900 MVA/RConn3 -- BG1/LConn3
  M2 900 MVA/RConn1 -- BG2/LConn1
  M2 900 MVA/RConn2 -- BG2/LConn2
  M2 900 MVA/RConn3 -- BG2/LConn3

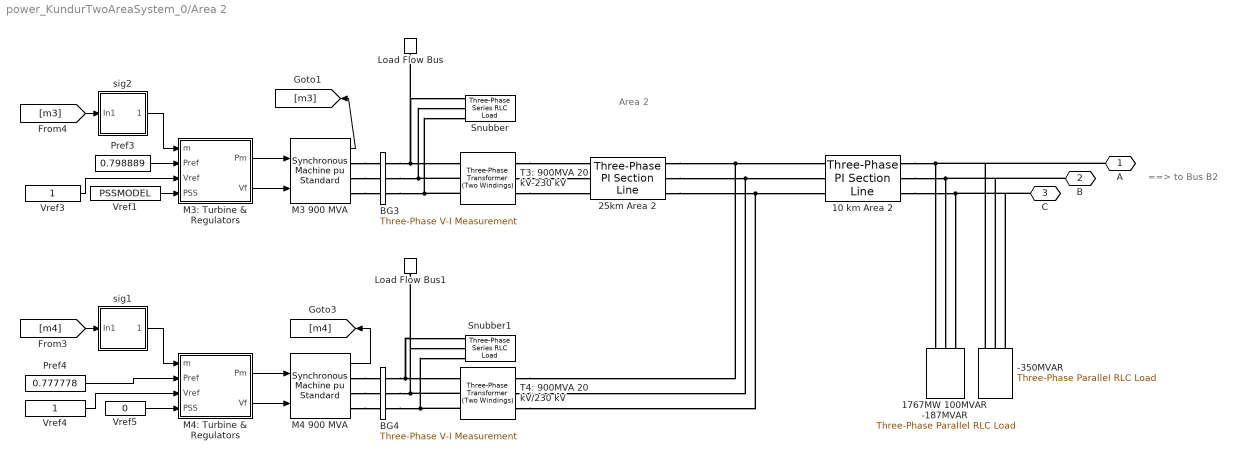
== system power_KundurTwoAreaSystem_0/Area 2 ==
  note: ==> to Bus B2
  note: Area 2
  -350MVAR : spsThreePhaseParallelRLCLoadLib/Three-Phase Parallel RLC Load  LConnTagsString=A|B|C  Configuration=Y (grounded)  NominalVoltage=230e3  Vabc=[1e3 1e3 1e3]  Vabcp=[1e3 1e3 1e3]  NominalFrequency=60  UnbalancedPower=off  ActivePower=0  InductivePower=0  CapacitivePower=350e6  Pabc=[10e3 9e3 11e3]  QLabc=[100 90 110]  QCabc=[100 90 110]  Pabcp=[10e3 9e3 11e3]  QLabcp=[100 90 110]  QCabcp=[100 90 110]  Measurements=None  LoadType=constant Z
  10 km Area 2 : spsThreePhasePISectionLineLib/Three-Phase PI Section Line  LConnTagsString=a|b|c  RConnTagsString=A|B|C  Length=10  Frequency=60  Resistances=[0.0001*529 1.61]  Inductances=[0.001*529/(377) 0.0061]  Capacitances=[0.00175/529/(377) 5.2489e-9]
  1767MW 100MVAR -187MVAR : spsThreePhaseParallelRLCLoadLib/Three-Phase Parallel RLC Load  LConnTagsString=A|B|C  Configuration=Y (grounded)  NominalVoltage=230e3  Vabc=[1e3 1e3 1e3]  Vabcp=[1e3 1e3 1e3]  NominalFrequency=60  UnbalancedPower=off  ActivePower=1767e6  InductivePower=100e6  CapacitivePower=187e6  Pabc=[10e3 9e3 11e3]  QLabc=[100 90 110]  QCabc=[100 90 110]  Pabcp=[10e3 9e3 11e3]  QLabcp=[100 90 110]  QCabcp=[100 90 110]  Measurements=None  LoadType=constant Z
  25km Area 2 : spsThreePhasePISectionLineLib/Three-Phase PI Section Line  LConnTagsString=a|b|c  RConnTagsString=A|B|C  Length=25  Frequency=60  Resistances=[0.0001*529 1.61]  Inductances=[0.001*529/(377) 0.0061]  Capacitances=[0.00175/529/(377) 5.2489e-9]
  BG3 : spsThreePhaseVIMeasurementLib/Three-Phase V-I Measurement  VoltageMeasurement=no  SetLabelV=on  LabelV=Vabc_G3  Vpu=on  VpuLL=off  CurrentMeasurement=no  SetLabelI=on  LabelI=Iabc_G3  Ipu=on  Pbase=900e6  Vbase=20e3  OutputType=Complex  PhasorSimulation=off  PSBequivalent=0
  BG4 : spsThreePhaseVIMeasurementLib/Three-Phase V-I Measurement  VoltageMeasurement=no  SetLabelV=on  LabelV=Vabc_G4  Vpu=on  VpuLL=off  CurrentMeasurement=no  SetLabelI=on  LabelI=Iabc_G4  Ipu=on  Pbase=900e6  Vbase=20e3  OutputType=Complex  PhasorSimulation=off  PSBequivalent=0
  Load Flow Bus : spsLoadFlowBusLib/Load Flow Bus  LConnTagsString=a  Phases=single  Connectors=on one side  ID=M3_Area2  Vbase=20e3  Vref=1  Vangle=0  VLF=1  VLFb=1  VLFc=1  angleLF=-16.02  angleLFb=0  angleLFc=0
      settings: AttributesFormatString=%<ID>\n%<Vbase>V\n%<VLF>pu\n%<angleLF>deg.  SourceProductBaseCode=PS
  Load Flow Bus1 : spsLoadFlowBusLib/Load Flow Bus  LConnTagsString=a  Phases=single  Connectors=on one side  ID=M4_Area2  Vbase=20e3  Vref=1  Vangle=0  VLF=1  VLFb=1  VLFc=1  angleLF=-26.66  angleLFb=0  angleLFc=0
      settings: AttributesFormatString=%<ID>\n%<Vbase>V\n%<VLF>pu\n%<angleLF>deg.  SourceProductBaseCode=PS
  M3 900 MVA : spsSynchronousMachinepuStandardLib/Synchronous Machine pu Standard  PresetModel=No  MechanicalLoad=Mechanical power Pm  ShowDetailedParameters=on  RotorType=Round  Units=per unit standard parameters  MeasurementBus=off  NominalParameters="[900E6  20000   60 ]"  Reactances1=[1.8 .3 .25 1.7 .55 .25 .2]  Reactances2=[ 1.305, 0.296, 0.252, 0.474, 0.243, 0.18 ]  dAxisTimeConstants=Open-circuit  qAxisTimeConstants=Open-circuit  TimeConstants1=[]  TimeConstants2=[8 .03 .4 .05]  TimeConstants3=[]  TimeConstants4=[]  TimeConstants5=[ 1.01, 0.053, 0.1 ]  TimeConstants6=[]  TimeConstants7=[]  TimeConstants8=[]  StatorResistance=0.0025  Mechanical="[ 6.175 0  4]"  PolePairs=4  InitialConditions=[0 -56.3243 0.8041 0.8041 0.8041 -22.4087 -142.409 97.5913 1.85092]  SetSaturation=off  Saturation=[0.6404,0.7127,0.8441,0.9214,0.9956,1.082,1.19,1.316,1.457;0.7,0.7698,0.8872,0.9466,0.9969,1.046,1.1,1.151,1.201]  LoadFlowParameters=[1 719000000 0 0 0]  TsPowergui=0  TsBlock=-1  IterativeModel=Trapezoidal non iterative  IterativeDiscreteModel=Trapezoidal non iterative  BusType=PV  Pref=719000000  Qref=0  Qmin=-inf  Qmax=inf  PLF=0  QLF=0
      settings: SourceProductBaseCode=PS
  M3: Turbine & Regulators : Subsystem
  M4 900 MVA : spsSynchronousMachinepuStandardLib/Synchronous Machine pu Standard  PresetModel=No  MechanicalLoad=Mechanical power Pm  ShowDetailedParameters=on  RotorType=Round  Units=per unit standard parameters  MeasurementBus=off  NominalParameters="[900E6  20000   60 ]"  Reactances1=[1.8 .3 .25 1.7 .55 .25 .2]  Reactances2=[ 1.305, 0.296, 0.252, 0.474, 0.243, 0.18 ]  dAxisTimeConstants=Open-circuit  qAxisTimeConstants=Open-circuit  TimeConstants1=[]  TimeConstants2=[8 .03 .4 .05]  TimeConstants3=[]  TimeConstants4=[]  TimeConstants5=[ 1.01, 0.053, 0.1 ]  TimeConstants6=[]  TimeConstants7=[]  TimeConstants8=[]  StatorResistance=0.0025  Mechanical="[ 6.175 0  4]"  PolePairs=4  InitialConditions=[0 -67.7513 0.783185 0.783185 0.783185 -33.268 -153.268 86.732 1.82209]  SetSaturation=off  Saturation=[0.6404,0.7127,0.8441,0.9214,0.9956,1.082,1.19,1.316,1.457;0.7,0.7698,0.8872,0.9466,0.9969,1.046,1.1,1.151,1.201]  LoadFlowParameters=[1 700000000 0 0 0]  TsPowergui=0  TsBlock=-1  IterativeModel=Trapezoidal non iterative  IterativeDiscreteModel=Trapezoidal non iterative  BusType=PV  Pref=700000000  Qref=0  Qmin=-inf  Qmax=inf  PLF=0  QLF=0
      settings: SourceProductBaseCode=PS
  M4: Turbine & Regulators : Subsystem
  Pref3 : Constant  Value=0.798889
  Pref4 : Constant  Value=0.777778
  Snubber : spsThreePhaseSeriesRLCLoadLib/Three-Phase Series RLC Load  LConnTagsString=A|B|C  Configuration=Y (grounded)  NominalVoltage=20000  Vabc=[1e3 1e3 1e3]  Vabcp=[1e3 1e3 1e3]  NominalFrequency=60  UnbalancedPower=off  ActivePower=1e6  InductivePower=0  CapacitivePower=1e7  Pabc=[10e3 9e3 11e3]  QLabc=[100 90 110]  QCabc=[100 90 110]  Pabcp=[10e3 9e3 11e3]  QLabcp=[100 90 110]  QCabcp=[100 90 110]  Measurements=None  LoadType=constant Z
  Snubber1 : spsThreePhaseSeriesRLCLoadLib/Three-Phase Series RLC Load  LConnTagsString=A|B|C  Configuration=Y (grounded)  NominalVoltage=20000  Vabc=[1e3 1e3 1e3]  Vabcp=[1e3 1e3 1e3]  NominalFrequency=60  UnbalancedPower=off  ActivePower=1e6  InductivePower=0  CapacitivePower=1e7  Pabc=[10e3 9e3 11e3]  QLabc=[100 90 110]  QCabc=[100 90 110]  Pabcp=[10e3 9e3 11e3]  QLabcp=[100 90 110]  QCabcp=[100 90 110]  Measurements=None  LoadType=constant Z
  T3: 900MVA 20 kV-230 kV : spsThreePhaseTransformerTwoWindingsLib/Three-Phase Transformer (Two Windings)  Winding1Connection=Delta (D1)  Winding2Connection=Yg  CoreType=Three single-phase transformers  SetSaturation=off  Hysteresis=off  DataFile='hysteresis'  SetInitialFlux=off  Measurements=None  UNITS=pu  NominalPower="[ 900e6   60 ]"  Winding1="[ 20e3  1e-6   0  ]"  Winding2="[ 230e3  1e-6   0.15 ]"  Rm=500  Lm=500  L0=0.5  Saturation="[ 0,0  ;  0.005,1.2  ;  1.0,1.4 ]"  InitialFluxes=[ 0.8 , -0.8 , 0.7 ]  BreakLoop=off  DiscreteSolver=Trapezoidal iterative  DataType=off  TransfoNumber=0
  T4: 900MVA 20 kV/230 kV : spsThreePhaseTransformerTwoWindingsLib/Three-Phase Transformer (Two Windings)  Winding1Connection=Delta (D1)  Winding2Connection=Yg  CoreType=Three single-phase transformers  SetSaturation=off  Hysteresis=off  DataFile='hysteresis'  SetInitialFlux=off  Measurements=None  UNITS=pu  NominalPower=[ 900e6 60 ]  Winding1="[ 20e3 1e-6  0.0]"  Winding2=[ 230e3 1e-6 0.15]  Rm=500  Lm=500  L0=0.5  Saturation="[ 0,0  ;  0.005,1.2  ;  1.0,1.4 ]"  InitialFluxes=[ 0.8 , -0.8 , 0.7 ]  BreakLoop=off  DiscreteSolver=Trapezoidal iterative  DataType=off  TransfoNumber=0
  Vref1 : Constant  Value=PSSMODEL
  Vref3 : Constant
  Vref4 : Constant
  Vref5 : Constant  Value=0
  sig1 : Subsystem
  sig2 : Subsystem
  A : PMIOPort  Side=Left
  B : PMIOPort  Port=2  Side=Left
  C : PMIOPort  Port=3  Side=Left
  wires:
  Pref3/1 -> M3: Turbine & Regulators/2(Pref)
  Vref3/1 -> M3: Turbine & Regulators/3(Vref)
  Pref4/1 -> M4: Turbine & Regulators/2(Pref)
  Vref4/1 -> M4: Turbine & Regulators/3(Vref)
  Vref5/1 -> M4: Turbine & Regulators/4(PSS)
  M3 900 MVA/1 -> [m3]
  M4 900 MVA/1 -> [m4]
  sig2/1(Out1) -> M3: Turbine & Regulators/1(m)
  sig1/1(Out1) -> M4: Turbine & Regulators/1(m)
  [m4] -> sig1/1(In1)
  [m3] -> sig2/1(In1)
  Vref1/1 -> M3: Turbine & Regulators/4(PSS)
  M3: Turbine & Regulators/1(Pm) -> M3 900 MVA/1
  M3: Turbine & Regulators/2(Vf) -> M3 900 MVA/2
  M4: Turbine & Regulators/1(Pm) -> M4 900 MVA/1
  M4: Turbine & Regulators/2(Vf) -> M4 900 MVA/2
  connections:
  T3: 900MVA 20 kV-230 kV/LConn3 -- BG3/RConn3 -- Snubber/LConn3
  T3: 900MVA 20 kV-230 kV/LConn2 -- BG3/RConn2 -- Snubber/LConn2
  Snubber/LConn1 -- Load Flow Bus/LConn1 -- T3: 900MVA 20 kV-230 kV/LConn1 -- BG3/RConn1
  T3: 900MVA 20 kV-230 kV/RConn3 -- 25km Area 2/LConn3
  T4: 900MVA 20 kV/230 kV/LConn3 -- Snubber1/LConn3 -- BG4/RConn3
  T4: 900MVA 20 kV/230 kV/LConn2 -- Snubber1/LConn2 -- BG4/RConn2
  Snubber1/LConn1 -- Load Flow Bus1/LConn1 -- BG4/RConn1 -- T4: 900MVA 20 kV/230 kV/LConn1
  T3: 900MVA 20 kV-230 kV/RConn2 -- 25km Area 2/LConn2
  T3: 900MVA 20 kV-230 kV/RConn1 -- 25km Area 2/LConn1
  25km Area 2/RConn2 -- 10 km Area 2/LConn2 -- T4: 900MVA 20 kV/230 kV/RConn2
  25km Area 2/RConn1 -- 10 km Area 2/LConn1 -- T4: 900MVA 20 kV/230 kV/RConn1
  25km Area 2/RConn3 -- 10 km Area 2/LConn3 -- T4: 900MVA 20 kV/230 kV/RConn3
  M3 900 MVA/RConn1 -- BG3/LConn1
  M3 900 MVA/RConn2 -- BG3/LConn2
  M3 900 MVA/RConn3 -- BG3/LConn3
  M4 900 MVA/RConn1 -- BG4/LConn1
  M4 900 MVA/RConn2 -- BG4/LConn2
  M4 900 MVA/RConn3 -- BG4/LConn3
  10 km Area 2/RConn1 -- A/RConn1 -- -350MVAR/LConn1 -- 1767MW 100MVAR -187MVAR/LConn1
  10 km Area 2/RConn2 -- 1767MW 100MVAR -187MVAR/LConn2 -- -350MVAR/LConn2 -- B/RConn1
  10 km Area 2/RConn3 -- -350MVAR/LConn3 -- C/RConn1 -- 1767MW 100MVAR -187MVAR/LConn3

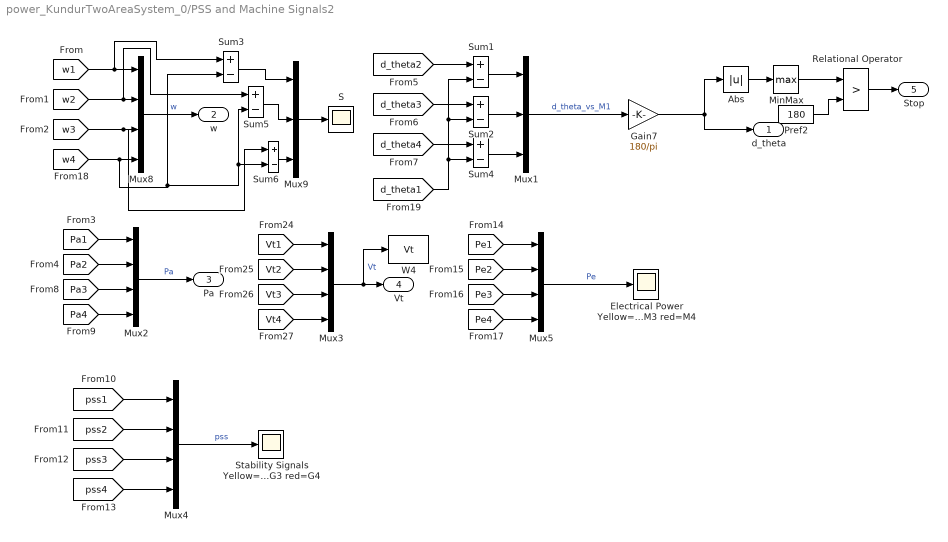
== system power_KundurTwoAreaSystem_0/PSS and Machine Signals2 ==
  Abs : Abs  SaturateOnIntegerOverflow=on
  "Electrical Power Yellow=M1 mag=M2 cyan=M3 red=M4 " : Scope
  Gain7 : Gain  Gain=180/pi
  MinMax : MinMax  Function=max  InputSameDT=on  SaturateOnIntegerOverflow=on
  Mux1 : Mux  Inputs=3
  Mux{2..5,8} (5 alike) : Mux
  Mux9 : Mux  Inputs=3
  Pref2 : Constant  Value=180
  Relational Operator : RelationalOperator  Operator=>  RndMeth=Nearest  InputSameDT=on
  S : Scope
  "Stability Signals Yellow=G1 mag=G2 cyan=G3 red=G4 " : Scope
  Sum{1..6} (6 alike) : Sum  Inputs=+-  InputSameDT=on  SaturateOnIntegerOverflow=on  OutDataTypeStr=Inherit: Same as first input
  W4 : ToWorkspace  VariableName=Vt  SampleTime=-1
  d_theta : Outport  VectorParamsAs1DForOutWhenUnconnected=off
  w : Outport  Port=2  VectorParamsAs1DForOutWhenUnconnected=off
  Pa : Outport  Port=3  VectorParamsAs1DForOutWhenUnconnected=off
  Vt : Outport  Port=4  VectorParamsAs1DForOutWhenUnconnected=off
  Stop : Outport  Port=5  VectorParamsAs1DForOutWhenUnconnected=off
  wires:
  [Pa1] -> Mux2/1
  Mux4/1 -> "Stability Signals Yellow=G1 mag=G2 cyan=G3 red=G4 "/1  "pss"
  [pss1] -> Mux4/1
  [pss2] -> Mux4/2
  [pss4] -> Mux4/4
  [pss3] -> Mux4/3
  Mux8/1 -> w/1  "w"
  Relational Operator/1 -> Stop/1
  Mux2/1 -> Pa/1  "Pa"
  [Pa2] -> Mux2/2
  [Pa3] -> Mux2/3
  [Pa4] -> Mux2/4
  [Vt1] -> Mux3/1
  [Vt2] -> Mux3/2
  [Vt3] -> Mux3/3
  [Vt4] -> Mux3/4
  Mux3/1 -> Vt/1, W4/1  "Vt"
  [Pe1] -> Mux5/1
  [Pe2] -> Mux5/2
  [Pe3] -> Mux5/3
  [Pe4] -> Mux5/4
  Mux5/1 -> "Electrical Power Yellow=M1 mag=M2 cyan=M3 red=M4 "/1  "Pe"
  [w1] -> Sum3/1, Mux8/1
  [w2] -> Sum5/1, Mux8/2
  [w3] -> Sum6/1, Mux8/3
  [w4] -> Sum3/2, Sum6/2, Sum5/2, Mux8/4
  Sum3/1 -> Mux9/1
  Sum5/1 -> Mux9/2
  Sum6/1 -> Mux9/3
  Mux9/1 -> S/1
  Mux1/1 -> Gain7/1  "d_theta_vs_M1"
  Abs/1 -> MinMax/1
  Pref2/1 -> Relational Operator/2
  MinMax/1 -> Relational Operator/1
  [d_theta2] -> Sum1/1
  Sum1/1 -> Mux1/1
  [d_theta3] -> Sum2/1
  [d_theta4] -> Sum4/1
  [d_theta1] -> Sum4/2, Sum2/2, Sum1/2
  Sum2/1 -> Mux1/2
  Sum4/1 -> Mux1/3
  Gain7/1 -> d_theta/1, Abs/1

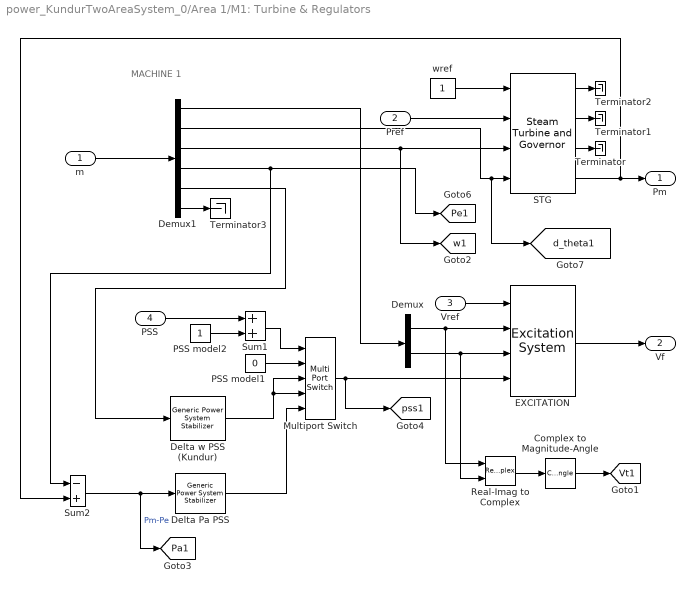
== system power_KundurTwoAreaSystem_0/Area 1/M1: Turbine & Regulators ==
  note: MACHINE 1
  m : Inport
  Pref : Inport  Port=2
  Vref : Inport  Port=3
  PSS : Inport  Port=4
  Complex to Magnitude-Angle : ComplexToMagnitudeAngle  Output=Magnitude
  Delta Pa PSS : spsGenericPowerSystemStabilizerLib/Generic Power System Stabilizer  Tsensor=15e-3  K=2.5*1.25  Twashout=1  Tleadlag1=[60e-3 1]  Tleadlag2=[0 0]  VSlimits=[-0.15 0.15]  Vinit=0  Plot_On=off  MagdB_On=on  FreqRange=logspace(-2,2,500)
      settings: SourceProductBaseCode=PS
  Delta w PSS (Kundur) : spsGenericPowerSystemStabilizerLib/Generic Power System Stabilizer  Tsensor=15e-3  K=30  Twashout=10  Tleadlag1=[50e-3 20e-3]  Tleadlag2=[3 5.4]  VSlimits=[-0.15 0.15]  Vinit=0  Plot_On=off  MagdB_On=on  FreqRange=logspace(-2,2,500)
      settings: SourceProductBaseCode=PS
  Demux : Demux  Outputs=2
      settings: DisplayOption=none
  Demux1 : Demux  Outputs=[2 1 1 1 1 1]
  EXCITATION : spsExcitationSystemLib/Excitation System  tr=20e-3  reg=[ 200, 0.001 ]  exc=[ 1, 0 ]  tgr=[ 0, 0 ]  damp=[ 0, 0 ]  sat=[ 0, 0 ]  lim=[-12.3 , 12.3, 0 ]  v0=[1,1.83395]
      settings: SourceProductBaseCode=PS
  Multiport Switch : MultiPortSwitch  Inputs=4  InputSameDT=on
  PSS model1 : Constant  Value=0
  PSS model2 : Constant
  Real-Imag to Complex : RealImagToComplex
  STG : spsSteamTurbineandGovernorLib/Steam Turbine and Governor  gentype=Tandem-compound (single mass)  reg1="[ 1  0.05    0 ]"  reg2="[ 0.001  0.15 ]"  reg3="[ -0.1  0.1  0  4.496 ]"  N=3600  turb1="[ 0  10   3.3   0.5   ]"  turb2="[   0   0.36    0.36   0.28   ]"  HA="[ 0.046  1.430  1.465   0.192 ]"  KA="[ 90.44  53.88  64.59   62.94  ]"  DA="[ 0.0115  0.3575  0.3663   0.0137  ]"  ini1=0.7778  ini2=[0.779316,-31.4247]
      settings: SourceProductBaseCode=PS
  Sum1 : Sum  InputSameDT=on  SaturateOnIntegerOverflow=on  OutDataTypeStr=Inherit: Same as first input
  Sum2 : Sum  Inputs=-+  InputSameDT=on  SaturateOnIntegerOverflow=on  OutDataTypeStr=Inherit: Same as first input
  Terminator{,1..3} (4 alike) : Terminator
  wref : Constant
  Pm : Outport  InitialOutput=0  VectorParamsAs1DForOutWhenUnconnected=off
  Vf : Outport  Port=2  InitialOutput=0  VectorParamsAs1DForOutWhenUnconnected=off
  tag scope: Pa1=global, Pe1=global, Vt1=global, d_theta1=global, pss1=global, w1=global
  wires:
  Demux/1 -> Real-Imag to Complex/1, EXCITATION/2
  Demux/2 -> Real-Imag to Complex/2, EXCITATION/3
  wref/1 -> STG/1
  Pref/1 -> STG/2
  m/1 -> Demux1/1
  Vref/1 -> EXCITATION/1
  Real-Imag to Complex/1 -> Complex to Magnitude-Angle/1
  EXCITATION/1 -> Vf/1
  Complex to Magnitude-Angle/1 -> [Vt1]
  Demux1/6 -> Terminator3/1
  PSS model1/1 -> Multiport Switch/2
  Delta w PSS (Kundur)/1 -> Multiport Switch/4, Multiport Switch/3
  Delta Pa PSS/1 -> Multiport Switch/5
  PSS model2/1 -> Sum1/2
  Sum1/1 -> Multiport Switch/1
  PSS/1 -> Sum1/1
  Demux1/1 -> Demux/1
  Demux1/3 -> [w1], STG/3
  Demux1/4 -> Sum2/1, [Pe1]
  Demux1/5 -> Delta w PSS (Kundur)/1
  Sum2/1 -> Delta Pa PSS/1, [Pa1]  "Pm-Pe"
  STG/3 -> Terminator/1
  Demux1/2 -> [d_theta1], STG/4
  STG/4 -> Pm/1, Sum2/2
  STG/2 -> Terminator1/1
  STG/1 -> Terminator2/1
  Multiport Switch/1 -> EXCITATION/4, [pss1]
